simulink subsystem "active_pacing_subsystem"  (R2020a)
settings: Solver=VariableStepAuto  StartTime=0.0  StopTime=10.0  RelTol=1e-3
libraries: frdmk64flib x1
settings Model: Creator=Ethan  LastModifiedBy=Ethan

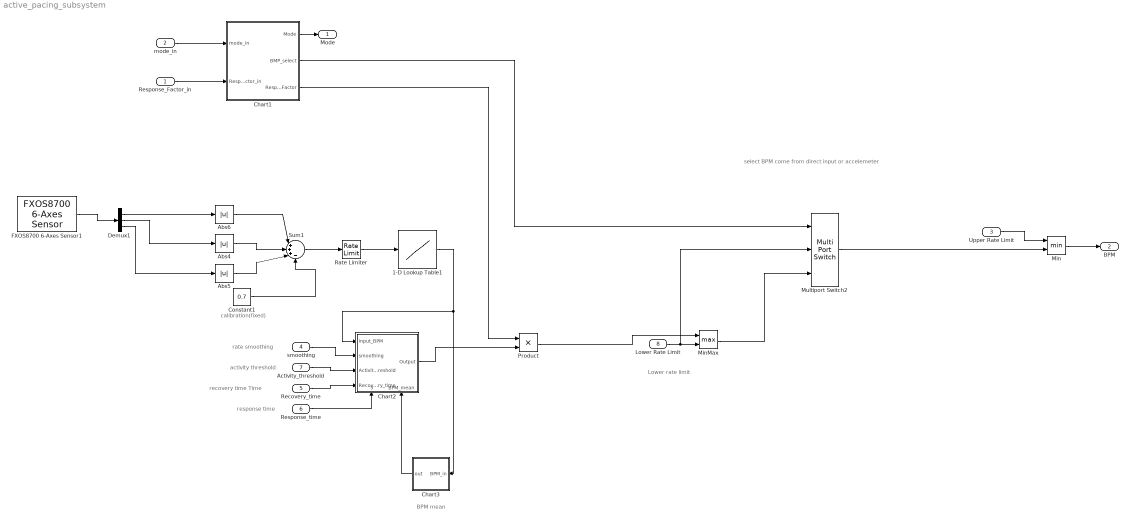
== system active_pacing_subsystem ==
  note: response time
  note: activity threshold
  note: calibration(fixed)
  note: rate smoothing
  note: recovery time Time
  note: BPM mean
  note: Lower rate limit
  note: select BPM come from direct input or accelemeter
  Response_Factor_in : Inport
  mode_in : Inport  Port=2
  Upper Rate Limit : Inport  Port=3
  smoothing : Inport  Port=4
  Recovery_time : Inport  Port=5
  Response_time : Inport  Port=6
  Activity_threshold : Inport  Port=7
  Lower Rate Limit : Inport  Port=8
  1-D Lookup Table1 : Lookup_n-D  NumberOfTableDimensions=1  BreakpointsForDimension1=[0:5]  Table=tanh([0:5])*175  InternalRulePriority=Speed  RndMeth=Simplest  InputSameDT=on
  Abs4 : Abs
  Abs5 : Abs
  Abs6 : Abs
  Chart1 : Stateflow chart  TreatAsAtomicUnit=on
  Chart2 : Stateflow chart  TreatAsAtomicUnit=on
      settings: PortSchema="{\"entries\":[{\"content\":{\"sides\":[{\"content\":{\"connectorIds\":[\"In2\",\"In4\",\"In3\",\"In1\"]},\"type\":\"ConnectorPlacement.EquallySpacedRectSide\",\"uuid\":\"702e1eeb-c8fc-4d4d-9b10-183ac648ac7c\"},{\"content\":{\"connectorIds\":[\"Out1\"],\"side\":\"RIGHT\"},\"type\":\"ConnectorPlacement.EquallySpacedRectSide\",\"uuid\":\"b30f496b-1ae7-4d8b-89a9-000fc18f8130\"},{\"content\":{\"connectorIds\":[],\"side\":\"TOP\"},\"type\":\"ConnectorPlacement.EquallySpacedRectSide\",\"uuid\":\"6f22146e-240a-4d3a-b228-c860f37f9cc9\"},{\"content\":{\"connectorIds\":[\"In5\",\"In6\"],\"side\":\"BOTTOM\"},\"type\":\"ConnectorPlacement.EquallySpacedRectSide\",\"uuid\":\"a6695b9c-9bdd-4dd8-a8cf-cc8c814be51a\"}]},\"type\":\"ConnectorPlacement.EquallySpacedConnector\",\"uuid\":\"5ce261cf-ddc8-4d93-ab97-81204610f659\"}],\"packageUris\":[\"http://schema.mathworks.com/mf0/Connector/19700101\"],\"version\":\"1.0\"}"
  Chart3 : Stateflow chart  TreatAsAtomicUnit=on
  Constant1 : Constant  Value=0.7
  Demux1 : Demux  Outputs=3
  FXOS8700 6-Axes Sensor1 : frdmk64flib/FXOS8700 6-Axes Sensor  Activesensor=Accelerometer only  ODR=800Hz  HybridODR=400Hz  Accelfullrange=-4g to +4g  SampleTime=-1
  Min : MinMax  Inputs=2
  MinMax : MinMax  Function=max  Inputs=2
  Multiport Switch2 : MultiPortSwitch  Inputs=2  DiagnosticForDefault=Warning
  Product : Product
  Rate Limiter : RateLimiter  SampleTimeMode=inherited
  Sum1 : Sum  Inputs=|+++-
  Mode : Outport
  BPM : Outport  Port=2
  wires:
  Abs4/1 -> Sum1/2
  Demux1/2 -> Abs4/1
  Recovery_time/1 -> Chart2/1(Recovery_time)
  Abs5/1 -> Sum1/3
  Sum1/1 -> Rate Limiter/1
  Chart3/1(out) -> Chart2/6(BPM_mean)
  Constant1/1 -> Sum1/4
  Abs6/1 -> Sum1/1
  1-D Lookup Table1/1 -> Chart2/2(input_BPM), Chart3/1(BPM_in)
  Product/1 -> MinMax/1
  Demux1/3 -> Abs5/1
  FXOS8700 6-Axes Sensor1/1 -> Demux1/1
  Response_Factor_in/1 -> Chart1/2(Response_Factor_in)
  Chart1/3(Response_Factor) -> Product/1
  mode_in/1 -> Chart1/1(mode_in)
  Chart1/2(BMP_select) -> Multiport Switch2/1
  Chart2/1(Output) -> Product/2
  Multiport Switch2/1 -> Min/2
  Rate Limiter/1 -> 1-D Lookup Table1/1
  Demux1/1 -> Abs6/1
  MinMax/1 -> Multiport Switch2/3
  Upper Rate Limit/1 -> Min/1
  Min/1 -> BPM/1
  Chart1/1(Mode) -> Mode/1
  Response_time/1 -> Chart2/5(Response_time)
  Lower Rate Limit/1 -> MinMax/2, Multiport Switch2/2
  smoothing/1 -> Chart2/4(smoothing)
  Activity_threshold/1 -> Chart2/3(Activity_threshold)

== stateflow chart active_pacing_subsystem/Chart3 ==
  state state3
    BPM_buffer = BPM_buffer + BPM_in;
  state state2
    BPM_buffer = BPM_buffer + BPM_in;
  state state1
    BPM_buffer = BPM_in;
    out =BPM_buffer;
  state state4
    BPM_buffer = (BPM_buffer + BPM_in)/4;
  (default) -> state1
  state2 -> state3 : after(10,msec)
  state1 -> state2 : after(10,msec)
  state4 -> state1 : after(100,msec)
  state3 -> state4 : after(10,msec)
  data: out output; BPM_in input; BPM_buffer local

== stateflow chart active_pacing_subsystem/Chart1 ==
  state IDLE
    Mode = 0;
  state Nonadptive
    BMP_select = 1;
    Mode = mode_in;
  state Adptive
    BMP_select = 2;
    Response_Factor = Response_Factor_in/16;
    Mode = mode_in - 5;
  (default) -> IDLE
  IDLE -> Adptive [order 1] : [mode_in>5]
  IDLE -> Nonadptive [order 2] : [mode_in <=5 && mode_in > 0]
  Nonadptive -> IDLE : [mode_in >5]
  Adptive -> IDLE : [mode_in<=5]
  data: Mode output; mode_in input; BMP_select output; Response_Factor_in input; Response_Factor output

== stateflow chart active_pacing_subsystem/Chart2 ==
  state delay_update
    Output = current_BPM;
  state Response
    current_BPM = current_BPM + (1-smoothing);
    Output = current_BPM;
  note: smooth out change in bpm
  state state0
    Output = input_BPM;
    current_BPM = input_BPM ;
  note: BPM following the sensor
  state State1
    Output = current_BPM;
  state Recovery
    current_BPM = current_BPM - smoothing;
    Output = current_BPM;
  state delay_update2
    Output = current_BPM;
  delay_update -> state0 [order 1] : [current_BPM > BPM_mean]
  delay_update -> Response [order 2] : after(10,msec)
  Response -> delay_update
  State1 -> Response [order 2] : after(Response_time,sec)[current_BPM < BPM_mean-Activity_threshold ]
  (default) -> state0
  state0 -> State1 : [abs(input_BPM -BPM_mean) > (1-smoothing)*10 ]
  State1 -> Recovery [order 1] : after(Recovery_time*60,sec)[current_BPM > BPM_mean+Activity_threshold]
  delay_update2 -> state0 [order 1] : [current_BPM < BPM_mean ]
  delay_update2 -> Recovery [order 2] : after(10,msec)
  Recovery -> delay_update2
  data: Recovery_time input; input_BPM input; current_BPM local; Activity_threshold input; smoothing input; Output output; Response_time input; BPM_mean input
